simulink model "frequency_band_state_controller_sim"  (R2020b)
settings: Solver=VariableStepAuto  StartTime=0.0  StopTime=stop_time  RelTol=1e-3
InitFcn:
  | frequency_band_state_controller_sim_init
StopFcn:
  | frequency_band_state_controller_sim_stop
settings Model: Creator=t96f346  LastModifiedBy=conno

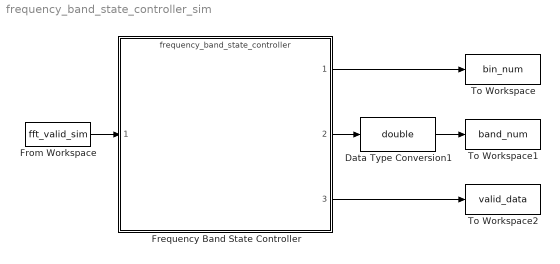
== system frequency_band_state_controller_sim ==
  Data Type Conversion1 : DataTypeConversion  OutDataTypeStr=double
  Frequency Band State Controller : ModelReference  ModelNameDialog=frequency_band_state_controller  SimulationMode=Normal  ModelReferenceVersion=2.34
  From Workspace : FromWorkspace  VariableName=fft_valid_sim  SampleTime=-1  Interpolate=off  OutputAfterFinalValue=Holding final value
  To Workspace : ToWorkspace  VariableName=bin_num  SampleTime=-1
      settings: Save2DSignal=2-D array (concatenate along first dimension)
  To Workspace1 : ToWorkspace  VariableName=band_num  SampleTime=-1
      settings: Save2DSignal=2-D array (concatenate along first dimension)
  To Workspace2 : ToWorkspace  VariableName=valid_data  SampleTime=-1
      settings: Save2DSignal=2-D array (concatenate along first dimension)
  wires:
  Frequency Band State Controller/1 -> To Workspace/1
  Frequency Band State Controller/2 -> Data Type Conversion1/1
  Frequency Band State Controller/3 -> To Workspace2/1
  From Workspace/1 -> Frequency Band State Controller/1
  Data Type Conversion1/1 -> To Workspace1/1
